simulink model "MRAS_Lyap"  (R2015a)
settings: Solver=ode4  StartTime=to  StopTime=tf  FixedStep=dt  RelTol=1e-3
values from neighbouring files (symbols this model uses):
  G = b/(s+a)    [MRAC_MIT2.m]
  gamma = 1    [MRAC_MIT2.m]
  k = 1    [MRAC_MIT2.m]
libraries: cstblocks x2
settings Model: Creator=dj  LastModifiedBy=dj

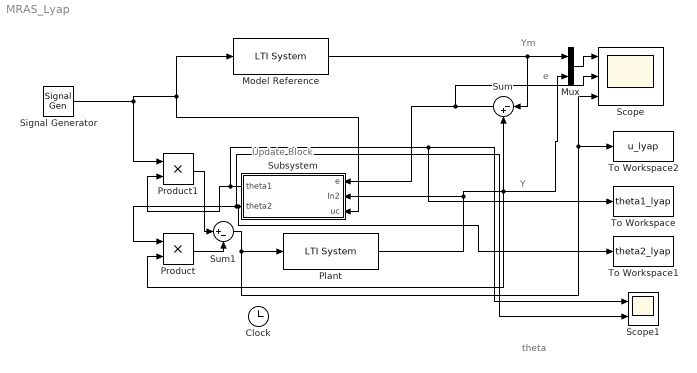
== system MRAS_Lyap ==
  note: e
  note: Y
  note: Ym
  note: theta
  note: Update Block
  Clock : Clock
  Model Reference : cstblocks/LTI System  sys=Gm  IC=[]
  Mux : Mux  Inputs=2
  Plant : cstblocks/LTI System  sys=k*G  IC=[]
  Product : Product
  Product1 : Product
  Scope : Scope  NumInputPorts=3
      settings: YMin=-5~-5~-5  YMax=5~5~5
  Scope1 : Scope  NumInputPorts=2
      settings: YMin=-5~-5  YMax=5~5
  Signal Generator : SignalGenerator  WaveForm=square  Frequency=0.05
  Subsystem : Subsystem
  Sum : Sum  Inputs=|-+
  Sum1 : Sum  Inputs=|+-
  To Workspace : ToWorkspace  VariableName=theta1_lyap  SaveFormat=Timeseries  SampleTime=-1
  To Workspace1 : ToWorkspace  VariableName=theta2_lyap  SaveFormat=Timeseries  SampleTime=-1
  To Workspace2 : ToWorkspace  VariableName=u_lyap  SaveFormat=Timeseries  SampleTime=-1
  wires:
  Model Reference/1 -> Mux/1, Sum/1
  Sum/1 -> Scope/2, Subsystem/1(e)
  Signal Generator/1 -> Model Reference/1, Subsystem/3(uc), Product1/1
  Plant/1 -> Product/2, Mux/2, Sum/2, Subsystem/2(In2)
  Mux/1 -> Scope/1
  Subsystem/1(theta1) -> To Workspace/1, Scope1/1, Product1/2
  Subsystem/2(theta2) -> Product/1, Scope1/2, To Workspace1/1
  Sum1/1 -> To Workspace2/1, Scope/3, Plant/1
  Product/1 -> Sum1/2
  Product1/1 -> Sum1/1

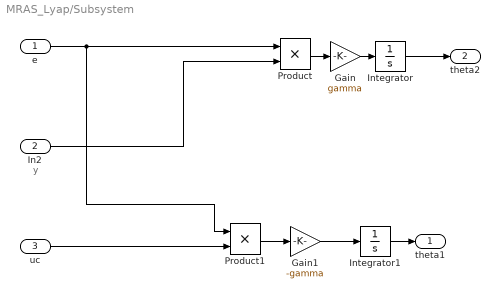
== system MRAS_Lyap/Subsystem ==
  note: y
  e : Inport
  In2 : Inport  Port=2
  uc : Inport  Port=3
  Gain : Gain  Gain=gamma
  Gain1 : Gain  Gain=-gamma
  Integrator : Integrator
  Integrator1 : Integrator
  Product : Product
  Product1 : Product
  theta1 : Outport
  theta2 : Outport  Port=2
  wires:
  e/1 -> Product/1, Product1/1
  Product/1 -> Gain/1
  Gain/1 -> Integrator/1
  Integrator/1 -> theta2/1
  uc/1 -> Product1/2
  Product1/1 -> Gain1/1
  Gain1/1 -> Integrator1/1
  Integrator1/1 -> theta1/1
  In2/1 -> Product/2
